simulink model "nlsimulink"  (R2024b)
settings: Solver=VariableStepAuto  StartTime=0.0  StopTime=300  FixedStep=1e-5
values from neighbouring files (symbols this model uses):
  A = [-1.166879465  -0.08802902616; 1.989203226 -2.349305992]    [TF_Linealizacion_Tanque.m]
  B = [0; 0.3]    [TF_Linealizacion_Tanque.m]
  C = [0 1]    [TF_Linealizacion_Tanque.m]
undefined symbols (not defined in the file or in its folder): CAi_ss, E1, E2, F, H, pCp, R, Tc_ss, Ti_ss, UA, V
libraries: slpidlib x3
settings Model: PacingRate=6  Creator=USER  LastModifiedBy=USER
settings DebuggingCC: UnderSpecifiedDimensionMsg=warning

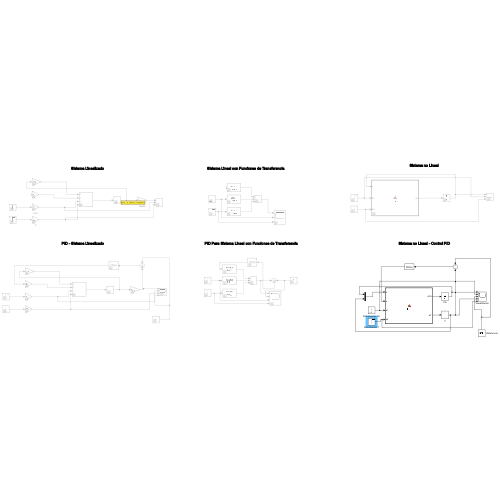
[thumbnail: Simulink's stored preview of the top-level diagram]
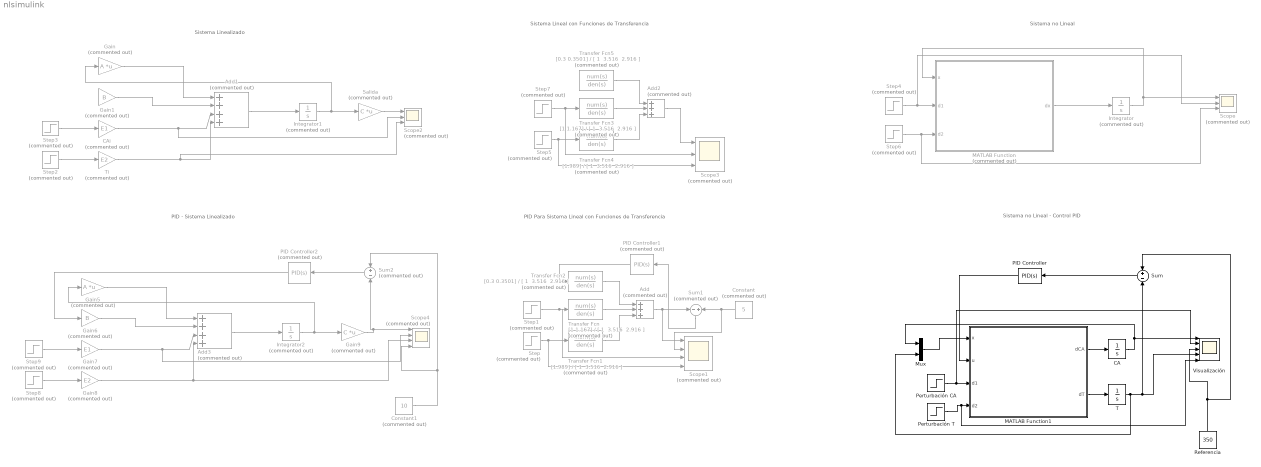
== system nlsimulink ==
  note: PID - Sistema Linealizado
  note: Sistema no Lineal - Control PID
  note: Sistema no Lineal
  note: Sistema Lineal con Funciones de Transferencia
  note: PID Para Sistema Lineal con Funciones de Transferencia
  note: Sistema Linealizado
  Add : Sum  Commented=on  Inputs=+++
  Add1 : Sum  Commented=on  Inputs=++++
  Add2 : Sum  Commented=on  Inputs=+++
  Add3 : Sum  Commented=on  Inputs=++++
  CA : Integrator  InitialCondition=8
  CAi : Gain  Commented=on  Gain=E1
  Constant : Constant  Commented=on  Value=5
  Constant1 : Constant  Commented=on  Value=10
  Gain : Gain  Commented=on  Gain=A  Multiplication=Matrix(K*u)
  Gain1 : Gain  Commented=on  Gain=B
  Gain5 : Gain  Commented=on  Gain=A  Multiplication=Matrix(K*u)
  Gain6 : Gain  Commented=on  Gain=B
  Gain7 : Gain  Commented=on  Gain=E1
  Gain8 : Gain  Commented=on  Gain=E2
  Gain9 : Gain  Commented=on  Gain=C  Multiplication=Matrix(K*u)
  Integrator : Integrator  Commented=on  InitialCondition=[8;300]
  Integrator1 : Integrator  Commented=on
  Integrator2 : Integrator  Commented=on
  MATLAB Function : MATLAB Function  Commented=on  TreatAsAtomicUnit=on
  MATLAB Function1 : MATLAB Function  TreatAsAtomicUnit=on
  Mux : Mux  Inputs=2
  PID Controller : slpidlib/PID Controller  Controller=PID  Form=Parallel  TimeDomain=Continuous-time  UseExternalTs=off  SampleTime=-1  IntegratorMethod=Forward Euler  FilterMethod=Forward Euler  ControllerParametersSource=internal  P=3  I=3  UseKiTs=off  D=2  UseExternalDerivativeSource=off  N=100  UseFilter=on  TunerSelectOption=Transfer Function Based (PID Tuner App)  InitialConditionSource=internal  InitialConditionForIntegrator=0  InitialConditionForFilter=0  DifferentiatorICPrevScaledInput=0  ExternalReset=none  TrackingMode=off  Kt=1  LimitOutput=off  SatLimitsSource=internal  UpperSaturationLimit=inf  LowerSaturationLimit=-inf  LinearizeAsGain=on  AntiWindupMode=none  Kb=1  LimitIntegrator=off  UpperIntegratorSaturationLimit=inf  LowerIntegratorSaturationLimit=-inf  POutMin=[]  POutMax=[]  IOutMin=[]  IOutMax=[]  DOutMin=[]  DOutMax=[]  NOutMin=[]  NOutMax=[]  SumOutMin=[]  SumOutMax=[]  SaturationOutMin=[]  SaturationOutMax=[]  PParamMin=[]  PParamMax=[]  IParamMin=[]  IParamMax=[]  DParamMin=[]  DParamMax=[]  NParamMin=[]  NParamMax=[]  KbParamMin=[]  KbParamMax=[]  KtParamMin=[]  KtParamMax=[]  KbOutMin=[]  KbOutMax=[]  KtOutMin=[]  KtOutMax=[]  IntegratorOutMin=[]  IntegratorOutMax=[]  FilterOutMin=[]  FilterOutMax=[]  SumI1OutMin=[]  SumI1OutMax=[]  SumI2OutMin=[]  SumI2OutMax=[]  SumI3OutMin=[]  SumI3OutMax=[]  SumI4OutMin=[]  SumI4OutMax=[]  SumDOutMin=[]  SumDOutMax=[]  DifferentiatorOutMin=[]  DifferentiatorOutMax=[]  FilterDiffOutCoefMin=[]  FilterDiffOutCoefMax=[]  ReciprocalOutMin=[]  ReciprocalOutMax=[]  SumDenOutMin=[]  SumDenOutMax=[]  SumNumOutMin=[]  SumNumOutMax=[]  DivideOutMin=[]  DivideOutMax=[]  UdiffTsProdOutMin=[]  UdiffTsProdOutMax=[]  NTsProdOutMin=[]  NTsProdOutMax=[]  UintegralTsProdOutMin=[]  UintegralTsProdOutMax=[]  UngainTsProdOutMin=[]  UngainTsProdOutMax=[]  ClampingZeroOutDataTypeStr=Inherit: Inherit via back propagation  ClampingZeroOutMin=[]  ClampingZeroOutMax=[]  FilterDenConstantOutDataTypeStr=Inherit: Inherit via back propagation  FilterDenConstantOutMin=[]  FilterDenConstantOutMax=[]  PCopyOutDataTypeStr=Inherit: Inherit via back propagation  PCopyOutMin=[]  PCopyOutMax=[]  NCopyOutDataTypeStr=Inherit: Inherit via back propagation  NCopyOutMin=[]  NCopyOutMax=[]  IntegratorContinuousStateAttributes=''  IntegratorStateMustResolveToSignalObject=off  IntegratorRTWStateStorageClass=Auto  FilterContinuousStateAttributes=''  FilterStateMustResolveToSignalObject=off  FilterRTWStateStorageClass=Auto  ParallelPVariant=InternalParameters  IdealPVariant=Disabled  IVariant=InternalParameters  DVariant=InternalParameters  IntegratorVariant=Continuous  SatVariant=Disabled  AWVariant=Passthrough  PCopyVariant=Disabled  TRVariant=Disabled  FdbkBlocksVariant=Forward  IdealPFdbkVariant=Disabled  SatFdbkVariant=Disabled  DerivativeFilterVariant=ContFilter  NVariant=InternalParameters  NCopyVariant=Disabled  FilterICVariant=InternalICsFilter  IntegratorICVariant=InternalICs  ExternalResetVariant=Disabled  TRSumVariant=Passthrough  SumFdbkVariant=Disabled  SumVariant=Sum_PID  TsampFilterVariant=InternalTs  TsampNgainVariant=Passthrough  TsampIntegralVariant=Disabled_SignalSpec  ExternalSaturationOutDataTypeStr=Inherit: Same as second input  DerivativeSourceVariant=ErrorSignal  PreIntVariant=InternalPreInt
  PID Controller1 : slpidlib/PID Controller  Commented=on  Controller=PID  Form=Parallel  TimeDomain=Continuous-time  UseExternalTs=off  SampleTime=-1  IntegratorMethod=Forward Euler  FilterMethod=Forward Euler  ControllerParametersSource=internal  P=1.5  I=1.5  UseKiTs=off  D=0  UseExternalDerivativeSource=off  N=100  UseFilter=on  TunerSelectOption=Transfer Function Based (PID Tuner App)  InitialConditionSource=internal  InitialConditionForIntegrator=0  InitialConditionForFilter=0  DifferentiatorICPrevScaledInput=0  ExternalReset=none  TrackingMode=off  Kt=1  LimitOutput=off  SatLimitsSource=internal  UpperSaturationLimit=inf  LowerSaturationLimit=-inf  LinearizeAsGain=on  AntiWindupMode=none  Kb=1  LimitIntegrator=off  UpperIntegratorSaturationLimit=inf  LowerIntegratorSaturationLimit=-inf  POutMin=[]  POutMax=[]  IOutMin=[]  IOutMax=[]  DOutMin=[]  DOutMax=[]  NOutMin=[]  NOutMax=[]  SumOutMin=[]  SumOutMax=[]  SaturationOutMin=[]  SaturationOutMax=[]  PParamMin=[]  PParamMax=[]  IParamMin=[]  IParamMax=[]  DParamMin=[]  DParamMax=[]  NParamMin=[]  NParamMax=[]  KbParamMin=[]  KbParamMax=[]  KtParamMin=[]  KtParamMax=[]  KbOutMin=[]  KbOutMax=[]  KtOutMin=[]  KtOutMax=[]  IntegratorOutMin=[]  IntegratorOutMax=[]  FilterOutMin=[]  FilterOutMax=[]  SumI1OutMin=[]  SumI1OutMax=[]  SumI2OutMin=[]  SumI2OutMax=[]  SumI3OutMin=[]  SumI3OutMax=[]  SumI4OutMin=[]  SumI4OutMax=[]  SumDOutMin=[]  SumDOutMax=[]  DifferentiatorOutMin=[]  DifferentiatorOutMax=[]  FilterDiffOutCoefMin=[]  FilterDiffOutCoefMax=[]  ReciprocalOutMin=[]  ReciprocalOutMax=[]  SumDenOutMin=[]  SumDenOutMax=[]  SumNumOutMin=[]  SumNumOutMax=[]  DivideOutMin=[]  DivideOutMax=[]  UdiffTsProdOutMin=[]  UdiffTsProdOutMax=[]  NTsProdOutMin=[]  NTsProdOutMax=[]  UintegralTsProdOutMin=[]  UintegralTsProdOutMax=[]  UngainTsProdOutMin=[]  UngainTsProdOutMax=[]  ClampingZeroOutDataTypeStr=Inherit: Inherit via back propagation  ClampingZeroOutMin=[]  ClampingZeroOutMax=[]  FilterDenConstantOutDataTypeStr=Inherit: Inherit via back propagation  FilterDenConstantOutMin=[]  FilterDenConstantOutMax=[]  PCopyOutDataTypeStr=Inherit: Inherit via back propagation  PCopyOutMin=[]  PCopyOutMax=[]  NCopyOutDataTypeStr=Inherit: Inherit via back propagation  NCopyOutMin=[]  NCopyOutMax=[]  IntegratorContinuousStateAttributes=''  IntegratorStateMustResolveToSignalObject=off  IntegratorRTWStateStorageClass=Auto  FilterContinuousStateAttributes=''  FilterStateMustResolveToSignalObject=off  FilterRTWStateStorageClass=Auto  ParallelPVariant=InternalParameters  IdealPVariant=Disabled  IVariant=InternalParameters  DVariant=InternalParameters  IntegratorVariant=Continuous  SatVariant=Disabled  AWVariant=Passthrough  PCopyVariant=Disabled  TRVariant=Disabled  FdbkBlocksVariant=Forward  IdealPFdbkVariant=Disabled  SatFdbkVariant=Disabled  DerivativeFilterVariant=ContFilter  NVariant=InternalParameters  NCopyVariant=Disabled  FilterICVariant=InternalICsFilter  IntegratorICVariant=InternalICs  ExternalResetVariant=Disabled  TRSumVariant=Passthrough  SumFdbkVariant=Disabled  SumVariant=Sum_PID  TsampFilterVariant=InternalTs  TsampNgainVariant=Passthrough  TsampIntegralVariant=Disabled_SignalSpec  ExternalSaturationOutDataTypeStr=Inherit: Same as second input  DerivativeSourceVariant=ErrorSignal  PreIntVariant=InternalPreInt
  PID Controller2 : slpidlib/PID Controller  Commented=on  Controller=PID  Form=Parallel  TimeDomain=Continuous-time  UseExternalTs=off  SampleTime=-1  IntegratorMethod=Forward Euler  FilterMethod=Forward Euler  ControllerParametersSource=internal  P=1  I=1  UseKiTs=off  D=0  UseExternalDerivativeSource=off  N=100  UseFilter=on  TunerSelectOption=Transfer Function Based (PID Tuner App)  InitialConditionSource=internal  InitialConditionForIntegrator=0  InitialConditionForFilter=0  DifferentiatorICPrevScaledInput=0  ExternalReset=none  TrackingMode=off  Kt=1  LimitOutput=off  SatLimitsSource=internal  UpperSaturationLimit=inf  LowerSaturationLimit=-inf  LinearizeAsGain=on  AntiWindupMode=none  Kb=1  LimitIntegrator=off  UpperIntegratorSaturationLimit=inf  LowerIntegratorSaturationLimit=-inf  POutMin=[]  POutMax=[]  IOutMin=[]  IOutMax=[]  DOutMin=[]  DOutMax=[]  NOutMin=[]  NOutMax=[]  SumOutMin=[]  SumOutMax=[]  SaturationOutMin=[]  SaturationOutMax=[]  PParamMin=[]  PParamMax=[]  IParamMin=[]  IParamMax=[]  DParamMin=[]  DParamMax=[]  NParamMin=[]  NParamMax=[]  KbParamMin=[]  KbParamMax=[]  KtParamMin=[]  KtParamMax=[]  KbOutMin=[]  KbOutMax=[]  KtOutMin=[]  KtOutMax=[]  IntegratorOutMin=[]  IntegratorOutMax=[]  FilterOutMin=[]  FilterOutMax=[]  SumI1OutMin=[]  SumI1OutMax=[]  SumI2OutMin=[]  SumI2OutMax=[]  SumI3OutMin=[]  SumI3OutMax=[]  SumI4OutMin=[]  SumI4OutMax=[]  SumDOutMin=[]  SumDOutMax=[]  DifferentiatorOutMin=[]  DifferentiatorOutMax=[]  FilterDiffOutCoefMin=[]  FilterDiffOutCoefMax=[]  ReciprocalOutMin=[]  ReciprocalOutMax=[]  SumDenOutMin=[]  SumDenOutMax=[]  SumNumOutMin=[]  SumNumOutMax=[]  DivideOutMin=[]  DivideOutMax=[]  UdiffTsProdOutMin=[]  UdiffTsProdOutMax=[]  NTsProdOutMin=[]  NTsProdOutMax=[]  UintegralTsProdOutMin=[]  UintegralTsProdOutMax=[]  UngainTsProdOutMin=[]  UngainTsProdOutMax=[]  ClampingZeroOutDataTypeStr=Inherit: Inherit via back propagation  ClampingZeroOutMin=[]  ClampingZeroOutMax=[]  FilterDenConstantOutDataTypeStr=Inherit: Inherit via back propagation  FilterDenConstantOutMin=[]  FilterDenConstantOutMax=[]  PCopyOutDataTypeStr=Inherit: Inherit via back propagation  PCopyOutMin=[]  PCopyOutMax=[]  NCopyOutDataTypeStr=Inherit: Inherit via back propagation  NCopyOutMin=[]  NCopyOutMax=[]  IntegratorContinuousStateAttributes=''  IntegratorStateMustResolveToSignalObject=off  IntegratorRTWStateStorageClass=Auto  FilterContinuousStateAttributes=''  FilterStateMustResolveToSignalObject=off  FilterRTWStateStorageClass=Auto  ParallelPVariant=InternalParameters  IdealPVariant=Disabled  IVariant=InternalParameters  DVariant=InternalParameters  IntegratorVariant=Continuous  SatVariant=Disabled  AWVariant=Passthrough  PCopyVariant=Disabled  TRVariant=Disabled  FdbkBlocksVariant=Forward  IdealPFdbkVariant=Disabled  SatFdbkVariant=Disabled  DerivativeFilterVariant=ContFilter  NVariant=InternalParameters  NCopyVariant=Disabled  FilterICVariant=InternalICsFilter  IntegratorICVariant=InternalICs  ExternalResetVariant=Disabled  TRSumVariant=Passthrough  SumFdbkVariant=Disabled  SumVariant=Sum_PID  TsampFilterVariant=InternalTs  TsampNgainVariant=Passthrough  TsampIntegralVariant=Disabled_SignalSpec  ExternalSaturationOutDataTypeStr=Inherit: Same as second input  DerivativeSourceVariant=ErrorSignal  PreIntVariant=InternalPreInt
  Perturbación CA : Step  Time=0  After=0  SampleTime=0
  Perturbación T : Step  Time=100  After=10  SampleTime=0
  Referencia : Constant  Value=350
  Salida : Gain  Commented=on  Gain=C  Multiplication=Matrix(K*u)
  Scope : Scope  Commented=on  NumInputPorts=3
  Scope1 : Scope  Commented=on  NumInputPorts=4
  Scope2 : Scope  Commented=on  NumInputPorts=3
  Scope3 : Scope  Commented=on  NumInputPorts=3
  Scope4 : Scope  Commented=on  NumInputPorts=4
  Step : Step  Commented=on  Time=150  SampleTime=0
  Step{1,4,6..7,9} (5 alike) : Step  Commented=on  Time=0  After=0  SampleTime=0
  Step2 : Step  Commented=on  Time=50  After=5  SampleTime=0
  Step3 : Step  Commented=on  Time=200  After=5  SampleTime=0
  Step5 : Step  Commented=on  Time=100  After=3  SampleTime=0
  Step8 : Step  Commented=on  Time=250  After=4  SampleTime=0
  Sum : Sum  Inputs=+-
  Sum1 : Sum  Commented=on  Inputs=-+
  Sum2 : Sum  Commented=on  Inputs=+-
  T : Integrator  InitialCondition=[8;300]
  Ti : Gain  Commented=on  Gain=E2
  Transfer Fcn : TransferFcn  Commented=on  Numerator=[1 1.167]  Denominator="[ 1  3.516  2.916 ]"
  Transfer Fcn1 : TransferFcn  Commented=on  Numerator=[1.989]  Denominator="[ 1  3.516  2.916 ]"
  Transfer Fcn2 : TransferFcn  Commented=on  Numerator=[0.3 0.3501]  Denominator="[ 1  3.516  2.916 ]"
  Transfer Fcn3 : TransferFcn  Commented=on  Numerator=[1 1.167]  Denominator="[ 1  3.516  2.916 ]"
  Transfer Fcn4 : TransferFcn  Commented=on  Numerator=[1.989]  Denominator="[ 1  3.516  2.916 ]"
  Transfer Fcn5 : TransferFcn  Commented=on  Numerator=[0.3 0.3501]  Denominator="[ 1  3.516  2.916 ]"
  Visualización : Scope  NumInputPorts=5
  wires:
  Integrator/1 -> Scope/1, MATLAB Function/1(x)
  Add/1 -> Scope1/1, Sum1/1
  Step/1 -> Scope1/4, Transfer Fcn1/1
  Integrator1/1 -> Gain/1, Salida/1
  Step3/1 -> CAi/1
  Step2/1 -> Ti/1
  Add1/1 -> Integrator1/1
  CAi/1 -> Scope2/2, Add1/3
  Ti/1 -> Scope2/3, Add1/4
  Gain1/1 -> Add1/2
  Gain/1 -> Add1/1
  PID Controller1/1 -> Transfer Fcn2/1
  Sum1/1 -> PID Controller1/1
  Transfer Fcn2/1 -> Add/1
  Transfer Fcn/1 -> Add/2
  Salida/1 -> Scope2/1
  Constant/1 -> Scope1/2, Sum1/2
  Step1/1 -> Scope1/3, Transfer Fcn/1
  Transfer Fcn1/1 -> Add/3
  MATLAB Function/1(dx) -> Integrator/1
  Step4/1 -> Scope/2, MATLAB Function/2(d1)
  Step6/1 -> Scope/3, MATLAB Function/3(d2)
  Perturbación CA/1 -> Visualización/2, MATLAB Function1/3(d1)
  Perturbación T/1 -> Visualización/5, MATLAB Function1/4(d2)
  MATLAB Function1/2(dT) -> T/1
  PID Controller/1 -> MATLAB Function1/2(u)
  Sum/1 -> PID Controller/1
  T/1 -> Sum/2, Visualización/4, Mux/2
  Referencia/1 -> Visualización/3, Sum/1
  MATLAB Function1/1(dCA) -> CA/1
  Mux/1 -> MATLAB Function1/1(x)
  CA/1 -> Visualización/1, Mux/1
  Transfer Fcn4/1 -> Add2/3
  Step5/1 -> Scope3/3, Transfer Fcn4/1
  Step7/1 -> Scope3/2, Transfer Fcn3/1
  Transfer Fcn3/1 -> Add2/2
  Transfer Fcn5/1 -> Add2/1
  Add2/1 -> Scope3/1
  Add3/1 -> Integrator2/1
  Gain5/1 -> Add3/1
  Step9/1 -> Gain7/1
  Gain9/1 -> Sum2/2, Scope4/1
  Gain8/1 -> Scope4/3, Add3/4
  Step8/1 -> Gain8/1
  Gain6/1 -> Add3/2
  Gain7/1 -> Scope4/2, Add3/3
  Integrator2/1 -> Gain5/1, Gain9/1
  PID Controller2/1 -> Gain6/1
  Sum2/1 -> PID Controller2/1
  Constant1/1 -> Sum2/1, Scope4/4

== matlab function nlsimulink/MATLAB Function1 ==
  data: dCA output; x input; u input; F parameter; V parameter; R parameter; E parameter; A parameter; H parameter; pCp parameter; CAi_ss parameter; Ti_ss parameter; UA parameter; dT output; d1 input; d2 input
function [dCA,dT]=fcn(x,u,F,V, R, E, A, H, pCp, CAi_ss, Ti_ss, UA,d1,d2)

k = A .* exp(-E ./ (R .* x(2)));
dCA = (F/V) * (CAi_ss+d1 - x(1)) - (k .* x(1));
dT = (F/V)*(Ti_ss+d2 - x(2)) + (-H/pCp).*k.* x(1) + (UA/(V*pCp))*(u - x(2));


end

== matlab function nlsimulink/MATLAB Function ==
  data: x input; F parameter; V parameter; R parameter; E parameter; A parameter; H parameter; pCp parameter; CAi_ss parameter; Ti_ss parameter; Tc_ss parameter; UA parameter; dx output; d1 input; d2 input
function dx = fcn(x, F, V, R, E, A, H, pCp, CAi_ss, Ti_ss, Tc_ss, UA,d1,d2)

k = A .* exp(-E ./ (R .* x(2)));
dx1 = (F/V) * (CAi_ss+d1 - x(1)) - (k .* x(1));
dx2 = (F/V)*(Ti_ss+d2 - x(2)) + (-H/pCp).*k.* x(1) + (UA/(V*pCp))*(Tc_ss - x(2));

dx=[dx1;dx2];


end
